simulink model "es3_sim"  (Simulink 7.5)
settings: Solver=ode45  StartTime=0.0  StopTime=10.0  RelTol=1e-3
values from neighbouring files (symbols this model uses):
  e_ = 0.1    [es3.m]
  epsilon2 = 10    [es3.m]
  p = 0.2    [es3.m]
settings Model: Creator=ceco-sciallo  LastModifiedBy=ceco-sciallo

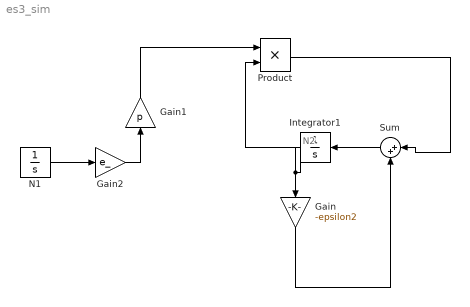
== system es3_sim ==
  note: N2
  Gain : Gain  Gain=-epsilon2  ParameterDataType=fixdt(1, 16)  ParameterScaling=2^0  OutDataType=fixdt(1, 16)  OutScaling=2^0
  Gain1 : Gain  Gain=p  ParameterDataType=fixdt(1, 16)  ParameterScaling=2^0  OutDataType=fixdt(1, 16)  OutScaling=2^0
  Gain2 : Gain  Gain=e_  ParameterDataType=fixdt(1, 16)  ParameterScaling=2^0  OutDataType=fixdt(1, 16)  OutScaling=2^0
  Integrator1 : Integrator
  N1 : Integrator
  Product : Product  OutDataType=fixdt(1, 16)  OutScaling=2^0  RndMeth=Zero
  Sum : Sum  Inputs=|++  OutDataType=fixdt(1, 16)  OutScaling=2^0
  wires:
  Integrator1/1 -> Gain/1, Product/2
  Gain/1 -> Sum/2
  N1/1 -> Gain2/1
  Gain1/1 -> Product/1
  Gain2/1 -> Gain1/1
  Product/1 -> Sum/1
  Sum/1 -> Integrator1/1
